simulink model "templatePQVFreplay"  (R2019b)
settings: Solver=ode23t  StartTime=0  StopTime=dataSim(l).Time(end)  FixedStep=Ts
model workspace (MAT data in the model file):
  AC8B_test_sdosession : sldodialogs.data.SessionData (value not decoded)
  tp34291882_bceb_4da8_b486_81ba615ab517 = [0 0.0333333 0.0666667 0.1 0.1333334 0.1666667 0.2 0.2333333 0.2666666 0.2999999 0.3333332 0.3666665 ... (13500 elements, 2700x5)]
  tp5fd81924_c6b2_4820_a4c1_c746ac51258e : object (value not decoded)
  tp61e2f470_2812_498a_af75_e87b8b944307 = [0 0.0333333 0.0666667 0.1 0.1333334 0.1666667 0.2 0.2333333 0.2666666 0.2999999 0.3333332 0.3666665 ... (13500 elements, 2700x5)]
  tpfa3056f0_c430_45b3_969f_b76cef1498ad : object (value not decoded)
undefined symbols (not defined in the file): dataSim, Fnom, l, MBase, Psnubber, Rsnubber, sys, Vnom
libraries: modelLibrary x8, powerlib x4, powerlib_meascontrol x1, GenLib x1, ideal_source x1
(part 2 of 2)

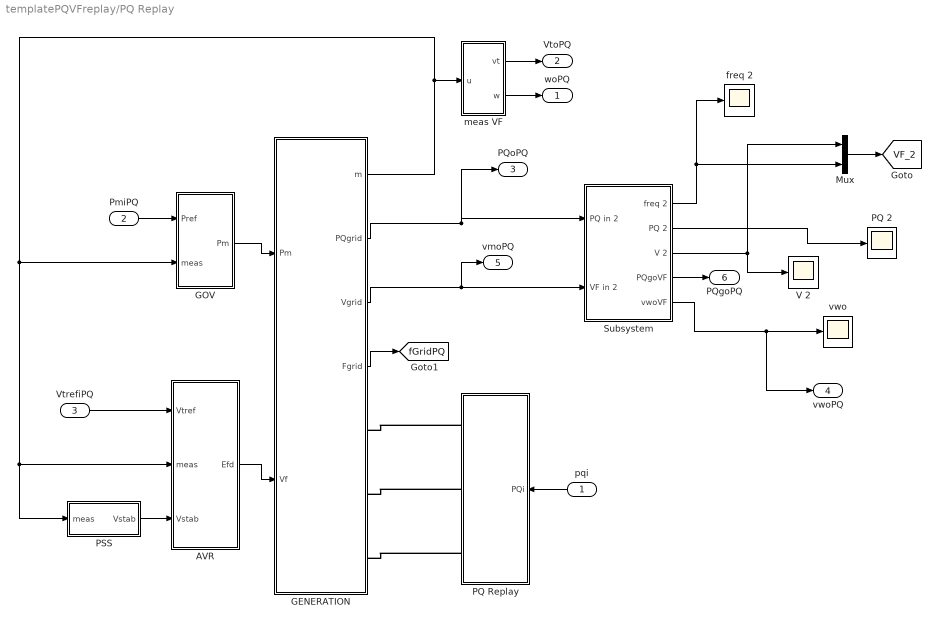
== system templatePQVFreplay/PQ Replay ==
  pqi : Inport  PortDimensions=2
  PmiPQ : Inport  Port=2
  VtrefiPQ : Inport  Port=3
  AVR : Subsystem  BlockChoice=ST4B
      link override ST4B: p=dyn.exst4b_31923_COLUSGT1
      settings: AttributesFormatString=%<BlockChoice>  TemplateBlock=modelLibrary/AVR  MemberBlocks=REXS,ST1A,ST4B
  GENERATION : Subsystem  BlockChoice=GENTPJ_TERMINAL
      link override GENROU_TERMINAL: g=sys.GENERATOR(1)  p=dyn.genrou_31923_COLUSGT1
      link override GENTPJ_TERMINAL: g=sys.GENERATOR(1)  p=dyn.genrou_31923_COLUSGT1
      settings: AttributesFormatString=%<BlockChoice>  TemplateBlock=modelLibrary/GENERATION  MemberBlocks=GENROU_TERMINAL,GENROU_TRANSFORMER,GENSAL_TRANSFORMER,GENTPJ_TERMINAL,GENTPJ_TRANSFORMER
  GOV : Subsystem  BlockChoice=GGOV1
      link override GGOV1: p=dyn.ggov1_31923_COLUSGT1  g=sys.GENERATOR(2)
      settings: AttributesFormatString=%<BlockChoice>  TemplateBlock=modelLibrary/GOV  MemberBlocks=GGOV1,IEEEG3
  Mux : Mux  Inputs=2
  PQ 2 : Scope
  PQ Replay : Subsystem  mask{Vrms=dataSim.Vact(1)*1e3, FreqHz=dataSim.Fact(1)}
      mask prompts: Vrms "Nominal LL Voltage (RMS)"; FreqHz "Frequency (Hz)"
  PSS : Subsystem  BlockChoice=PSS2B
      link override PSS2B: p=dyn.pss2b_31923_COLUSGT1
      link override PSS2B/Bus Selector3: OutputSignals="Mechanical.Rotor speed deviation  dw (pu),Mechanical.Electrical power  Pe (pu)"
      settings: AttributesFormatString=%<BlockChoice>  TemplateBlock=modelLibrary/PSS  MemberBlocks=PSS1A,PSS2A,PSS2B
  Subsystem : Subsystem
  V 2 : Scope
  freq 2 : Scope
  meas VF : Subsystem
  vwo : Scope
  woPQ : Outport
  VtoPQ : Outport  Port=2
  PQoPQ : Outport  Port=3  SampleTime=1/30
  vwoPQ : Outport  Port=4
  vmoPQ : Outport  Port=5
  PQgoPQ : Outport  Port=6  SampleTime=1/30
  tag scope: VF_2=global, fGridPQ=global
  wires:
  GENERATION/3(Vgrid) -> vmoPQ/1, Subsystem/2(VF in 2)
  GENERATION/1(m) -> GOV/2(meas), PSS/1(meas), AVR/2(meas), meas VF/1(u)
  GENERATION/2(PQgrid) -> PQoPQ/1, Subsystem/1(PQ in 2)
  meas VF/1(vt) -> VtoPQ/1
  meas VF/2(w) -> woPQ/1
  Subsystem/1(freq 2) -> Mux/2, freq 2/1
  Subsystem/2(PQ 2) -> PQ 2/1
  Subsystem/4(PQgoVF) -> PQgoPQ/1
  Subsystem/3(V 2) -> V 2/1, Mux/1
  Subsystem/5(vwoVF) -> vwoPQ/1, vwo/1
  PmiPQ/1 -> GOV/1(Pref)
  GOV/1(Pm) -> GENERATION/1(Pm)
  AVR/1(Efd) -> GENERATION/2(Vf)
  VtrefiPQ/1 -> AVR/1(Vtref)
  pqi/1 -> PQ Replay/1(PQi)
  PSS/1(Vstab) -> AVR/3(Vstab)
  Mux/1 -> [VF_2]
  GENERATION/4(Fgrid) -> [fGridPQ]
  connections:
  PQ Replay/RConn1 -- GENERATION/RConn1
  PQ Replay/RConn2 -- GENERATION/RConn2
  PQ Replay/RConn3 -- GENERATION/RConn3

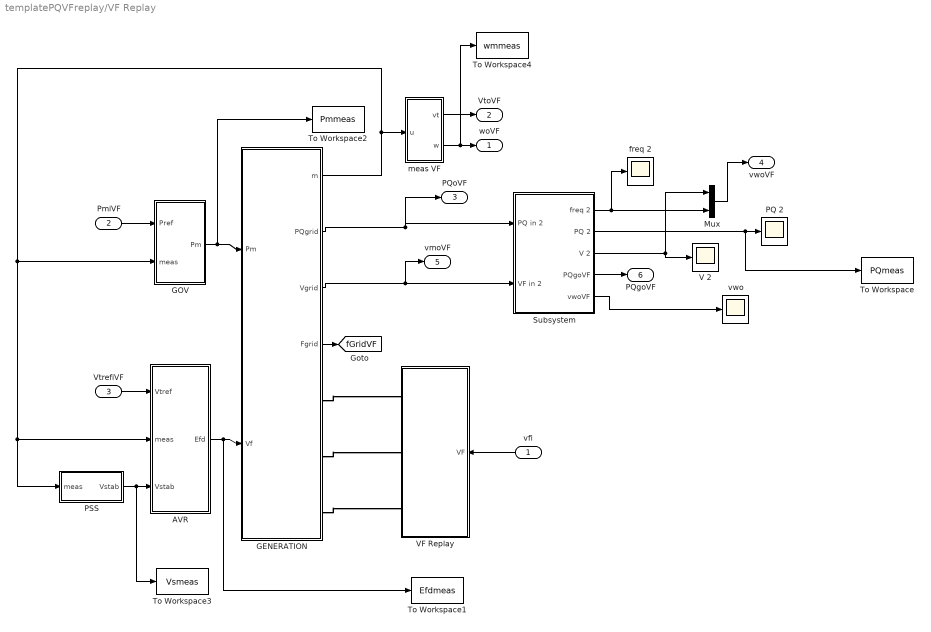
== system templatePQVFreplay/VF Replay ==
  vfi : Inport  PortDimensions=2
  PmiVF : Inport  Port=2
  VtrefiVF : Inport  Port=3
  AVR : Subsystem  BlockChoice=ST4B
      link override ST4B: p=dyn.exst4b_31923_COLUSGT1
      settings: AttributesFormatString=%<BlockChoice>  TemplateBlock=modelLibrary/AVR  MemberBlocks=REXS,ST1A,ST4B
  GENERATION : Subsystem  BlockChoice=GENTPJ_TERMINAL
      link override GENROU_TERMINAL: g=sys.GENERATOR(1)  p=dyn.genrou_31923_COLUSGT1
      link override GENTPJ_TERMINAL: g=sys.GENERATOR(1)  p=dyn.genrou_31923_COLUSGT1
      settings: AttributesFormatString=%<BlockChoice>  TemplateBlock=modelLibrary/GENERATION  MemberBlocks=GENROU_TERMINAL,GENROU_TRANSFORMER,GENSAL_TRANSFORMER,GENTPJ_TERMINAL,GENTPJ_TRANSFORMER
  GOV : Subsystem  BlockChoice=GGOV1
      link override GGOV1: p=dyn.ggov1_31923_COLUSGT1  g=sys.GENERATOR(2)
      settings: AttributesFormatString=%<BlockChoice>  TemplateBlock=modelLibrary/GOV  MemberBlocks=GGOV1,IEEEG3
  Mux : Mux  Inputs=2
  PQ 2 : Scope
  PSS : Subsystem  BlockChoice=PSS2B
      link override PSS2B: p=dyn.pss2b_31923_COLUSGT1
      link override PSS2B/Bus Selector3: OutputSignals="Mechanical.Rotor speed deviation  dw (pu),Mechanical.Electrical power  Pe (pu)"
      settings: AttributesFormatString=%<BlockChoice>  TemplateBlock=modelLibrary/PSS  MemberBlocks=PSS1A,PSS2A,PSS2B
  Subsystem : Subsystem
  To Workspace : ToWorkspace  VariableName=PQmeas  SampleTime=1/60
  To Workspace1 : ToWorkspace  VariableName=Efdmeas  SampleTime=1/60
  To Workspace2 : ToWorkspace  VariableName=Pmmeas  SampleTime=1/60
  To Workspace3 : ToWorkspace  VariableName=Vsmeas  SampleTime=1/60
  To Workspace4 : ToWorkspace  VariableName=wmmeas  SampleTime=1/60
  V 2 : Scope
  VF Replay : Subsystem
  freq 2 : Scope
  meas VF : Subsystem
  vwo : Scope
  woVF : Outport
  VtoVF : Outport  Port=2
  PQoVF : Outport  Port=3  SampleTime=1/30
  vwoVF : Outport  Port=4
  vmoVF : Outport  Port=5
  PQgoVF : Outport  Port=6  SampleTime=1/30
  tag scope: fGridVF=global
  wires:
  GENERATION/3(Vgrid) -> vmoVF/1, Subsystem/2(VF in 2)
  GENERATION/2(PQgrid) -> PQoVF/1, Subsystem/1(PQ in 2)
  meas VF/1(vt) -> VtoVF/1
  Subsystem/1(freq 2) -> freq 2/1, Mux/2
  Subsystem/2(PQ 2) -> To Workspace/1, PQ 2/1
  Subsystem/4(PQgoVF) -> PQgoVF/1
  Subsystem/3(V 2) -> V 2/1, Mux/1
  Subsystem/5(vwoVF) -> vwo/1
  Mux/1 -> vwoVF/1
  PmiVF/1 -> GOV/1(Pref)
  GOV/1(Pm) -> To Workspace2/1, GENERATION/1(Pm)
  PSS/1(Vstab) -> To Workspace3/1, AVR/3(Vstab)
  AVR/1(Efd) -> To Workspace1/1, GENERATION/2(Vf)
  VtrefiVF/1 -> AVR/1(Vtref)
  vfi/1 -> VF Replay/1(VF)
  GENERATION/1(m) -> GOV/2(meas), PSS/1(meas), AVR/2(meas), meas VF/1(u)
  meas VF/2(w) -> To Workspace4/1, woVF/1
  GENERATION/4(Fgrid) -> [fGridVF]
  connections:
  GENERATION/RConn1 -- VF Replay/RConn1
  GENERATION/RConn2 -- VF Replay/RConn2
  GENERATION/RConn3 -- VF Replay/RConn3

== system templatePQVFreplay/view ==
  Gain : Gain  Gain=1/MBase
  Selector2 : Selector  InputPortWidth=4  IndexOptions=Index vector (dialog)  Indices=[2 4]  OutputSizes=1
  Selector3 : Selector  InputPortWidth=4  IndexOptions=Index vector (dialog)  Indices=[1 3]  OutputSizes=1
  P : Outport
  Q : Outport  Port=2
  wires:
  [PQ_2] -> Gain/1
  Gain/1 -> Selector2/1, Selector3/1
  Selector2/1 -> Q/1
  Selector3/1 -> P/1

== system templatePQVFreplay/view1 ==
  Gain : Gain
  Selector2 : Selector  InputPortWidth=4  IndexOptions=Index vector (dialog)  Indices=[3 4]  OutputSizes=1
  Selector3 : Selector  InputPortWidth=4  IndexOptions=Index vector (dialog)  Indices=[1 2]  OutputSizes=1
  V : Outport
  F : Outport  Port=2
  wires:
  [VF_2] -> Gain/1
  Gain/1 -> Selector2/1, Selector3/1
  Selector2/1 -> F/1
  Selector3/1 -> V/1

== system templatePQVFreplay/PQ Replay/AVR ==
  Vtref : Inport
  meas : Inport  Port=2
  Vstab : Inport  Port=3
  ST4B : modelLibrary/ST4B  p=dyn.exst4b_31923_COLUSGT1
  Efd : Outport
  wires:
  Vtref/1 -> ST4B/1
  meas/1 -> ST4B/2
  Vstab/1 -> ST4B/3
  ST4B/1 -> Efd/1

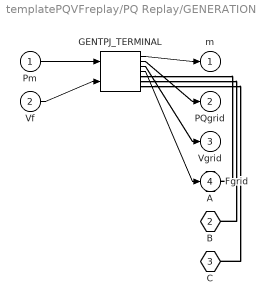
== system templatePQVFreplay/PQ Replay/GENERATION ==
  Pm : Inport
  Vf : Inport  Port=2
  GENTPJ_TERMINAL : modelLibrary/GENTPJ_TERMINAL  g=sys.GENERATOR(1)  p=dyn.genrou_31923_COLUSGT1
  A : PMIOPort  Side=Right
  B : PMIOPort  Port=2  Side=Right
  C : PMIOPort  Port=3  Side=Right
  m : Outport
  PQgrid : Outport  Port=2
  Vgrid : Outport  Port=3
  Fgrid : Outport  Port=4
  wires:
  Pm/1 -> GENTPJ_TERMINAL/1
  Vf/1 -> GENTPJ_TERMINAL/2
  GENTPJ_TERMINAL/1 -> m/1
  GENTPJ_TERMINAL/2 -> PQgrid/1
  GENTPJ_TERMINAL/3 -> Vgrid/1
  GENTPJ_TERMINAL/4 -> Fgrid/1
  connections:
  GENTPJ_TERMINAL/RConn1 -- A/RConn1
  GENTPJ_TERMINAL/RConn2 -- B/RConn1
  GENTPJ_TERMINAL/RConn3 -- C/RConn1

== system templatePQVFreplay/PQ Replay/GOV ==
  Pref : Inport
  meas : Inport  Port=2
  GGOV1 : modelLibrary/GGOV1  p=dyn.ggov1_31923_COLUSGT1  g=sys.GENERATOR(2)
  Pm : Outport
  wires:
  Pref/1 -> GGOV1/1
  meas/1 -> GGOV1/2
  GGOV1/1 -> Pm/1

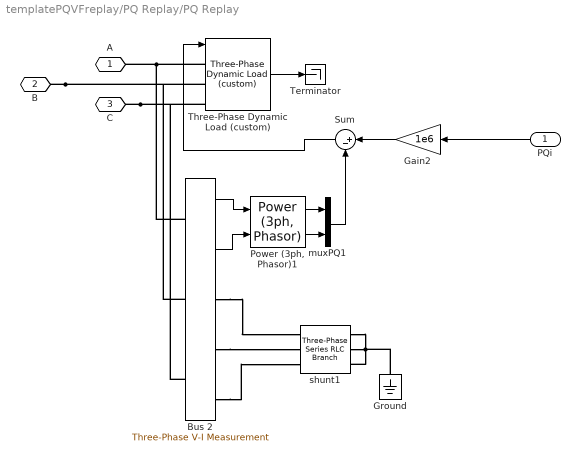
== system templatePQVFreplay/PQ Replay/PQ Replay ==
  PQi : Inport
  Bus 2 : powerlib/Measurements/Three-Phase V-I Measurement  VoltageMeasurement=phase-to-ground  SetLabelV=off  LabelV=Vabc  Vpu=off  VpuLL=off  CurrentMeasurement=yes  SetLabelI=off  LabelI=Iabc  Ipu=off  Pbase=100e6  Vbase=500e3  OutputType=Complex  PhasorSimulation=on  PSBequivalent=0
      settings: SourceProductName=Simscape Electrical
  Gain2 : Gain  Gain=1e6
  Ground : powerlib/Elements/Ground  LConnTagsString=a
      settings: SourceProductName=Simscape Electrical
  "Power (3ph, Phasor)1" : powerlib_meascontrol/Measurements/Power (3ph, Phasor)
      settings: SourceProductName=Simscape Electrical  SourceProductBaseCode=PS
  Sum : Sum  Inputs=|+-
  Terminator : Terminator
  Three-Phase Dynamic Load (custom) : GenLib/Three-Phase Dynamic Load (custom)  NominalVoltage=[ Vrms FreqHz ]  ActiveReactivePowers="[-dataSim.Pact(1)-Psnubber/1e6  -dataSim.Qact(1)]*1e6"  PositiveSequence=[1 0]  ExternalControl=on  NpNq=[1.3 2]  TimeConstants="[0  0  0  0]"  MinimumVoltage=0.7  LoadFlowParameters=[4,0,0,0,0]
  muxPQ1 : Mux  Inputs=2
  shunt1 : powerlib/Elements/Three-Phase Series RLC Branch  LConnTagsString=A|B|C  RConnTagsString=A|B|C  BranchType=R  Resistance=Rsnubber  Inductance=1e-3  Capacitance=1e-6  Measurements=None
      settings: SourceProductName=Simscape Electrical
  A : PMIOPort  Side=Right
  B : PMIOPort  Port=2  Side=Right
  C : PMIOPort  Port=3  Side=Right
  wires:
  Three-Phase Dynamic Load (custom)/1 -> Terminator/1
  Bus 2/2 -> "Power (3ph, Phasor)1"/2
  Bus 2/1 -> "Power (3ph, Phasor)1"/1
  Sum/1 -> Three-Phase Dynamic Load (custom)/1
  "Power (3ph, Phasor)1"/2 -> muxPQ1/2
  Gain2/1 -> Sum/1
  "Power (3ph, Phasor)1"/1 -> muxPQ1/1
  PQi/1 -> Gain2/1
  muxPQ1/1 -> Sum/2
  connections:
  B/RConn1 -- Three-Phase Dynamic Load (custom)/LConn2 -- Bus 2/LConn2
  Bus 2/LConn1 -- Three-Phase Dynamic Load (custom)/LConn1 -- A/RConn1
  C/RConn1 -- Three-Phase Dynamic Load (custom)/LConn3 -- Bus 2/LConn3
  Bus 2/RConn1 -- shunt1/LConn1
  Bus 2/RConn2 -- shunt1/LConn2
  Bus 2/RConn3 -- shunt1/LConn3
  shunt1/RConn1 -- shunt1/RConn2 -- Ground/LConn1 -- shunt1/RConn3

== system templatePQVFreplay/PQ Replay/PSS ==
  meas : Inport
  PSS2B : modelLibrary/PSS2B  p=dyn.pss2b_31923_COLUSGT1
  Vstab : Outport
  wires:
  meas/1 -> PSS2B/1
  PSS2B/1 -> Vstab/1

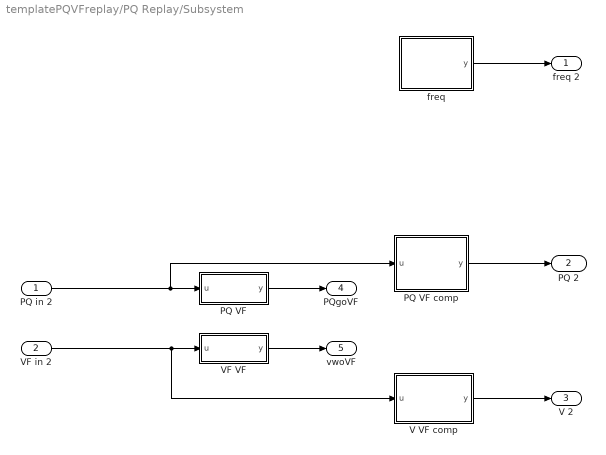
== system templatePQVFreplay/PQ Replay/Subsystem ==
  PQ in 2 : Inport
  VF in 2 : Inport  Port=2
  PQ VF : Subsystem
  PQ VF comp : Subsystem
  V VF comp : Subsystem
  VF VF : Subsystem
  freq : Subsystem
  freq 2 : Outport
  PQ 2 : Outport  Port=2
  V 2 : Outport  Port=3
  PQgoVF : Outport  Port=4
  vwoVF : Outport  Port=5
  wires:
  V VF comp/1(y) -> V 2/1
  VF in 2/1 -> V VF comp/1(u), VF VF/1(u)
  PQ VF comp/1("y ") -> PQ 2/1
  freq/1(y) -> freq 2/1
  PQ VF/1(y) -> PQgoVF/1
  VF VF/1(y) -> vwoVF/1
  PQ in 2/1 -> PQ VF/1(u), PQ VF comp/1(u)

== system templatePQVFreplay/PQ Replay/meas VF ==
  u : Inport
  Bus Selector6 : BusSelector  OutputSignals="dq0 components.Stator voltage  vd (pu),dq0 components.Stator voltage  vq (pu),Mechanical.Rotor speed  wm  (pu)"
  Euclidian Norm5 : Subsystem
  wo PQ : Subsystem
  vt : Outport
  w : Outport  Port=2
  wires:
  u/1 -> Bus Selector6/1
  Bus Selector6/2 -> Euclidian Norm5/2(u2)  "<Stator voltage  vq (pu)>"
  Bus Selector6/1 -> Euclidian Norm5/1(u1)  "<Stator voltage  vd (pu)>"
  Euclidian Norm5/1(y) -> vt/1  "vt"
  Bus Selector6/3 -> wo PQ/1(u)  "<Rotor speed  wm  (pu)>"
  wo PQ/1(y) -> w/1

== system templatePQVFreplay/VF Replay/AVR ==
  Vtref : Inport
  meas : Inport  Port=2
  Vstab : Inport  Port=3
  ST4B : modelLibrary/ST4B  p=dyn.exst4b_31923_COLUSGT1
  Efd : Outport
  wires:
  Vtref/1 -> ST4B/1
  meas/1 -> ST4B/2
  Vstab/1 -> ST4B/3
  ST4B/1 -> Efd/1

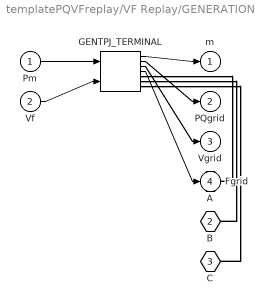
== system templatePQVFreplay/VF Replay/GENERATION ==
  Pm : Inport
  Vf : Inport  Port=2
  GENTPJ_TERMINAL : modelLibrary/GENTPJ_TERMINAL  g=sys.GENERATOR(1)  p=dyn.genrou_31923_COLUSGT1
  A : PMIOPort  Side=Right
  B : PMIOPort  Port=2  Side=Right
  C : PMIOPort  Port=3  Side=Right
  m : Outport
  PQgrid : Outport  Port=2
  Vgrid : Outport  Port=3
  Fgrid : Outport  Port=4
  wires:
  Pm/1 -> GENTPJ_TERMINAL/1
  Vf/1 -> GENTPJ_TERMINAL/2
  GENTPJ_TERMINAL/1 -> m/1
  GENTPJ_TERMINAL/2 -> PQgrid/1
  GENTPJ_TERMINAL/3 -> Vgrid/1
  GENTPJ_TERMINAL/4 -> Fgrid/1
  connections:
  GENTPJ_TERMINAL/RConn1 -- A/RConn1
  GENTPJ_TERMINAL/RConn2 -- B/RConn1
  GENTPJ_TERMINAL/RConn3 -- C/RConn1

== system templatePQVFreplay/VF Replay/GOV ==
  Pref : Inport
  meas : Inport  Port=2
  GGOV1 : modelLibrary/GGOV1  p=dyn.ggov1_31923_COLUSGT1  g=sys.GENERATOR(2)
  Pm : Outport
  wires:
  Pref/1 -> GGOV1/1
  meas/1 -> GGOV1/2
  GGOV1/1 -> Pm/1

== system templatePQVFreplay/VF Replay/PSS ==
  meas : Inport
  PSS2B : modelLibrary/PSS2B  p=dyn.pss2b_31923_COLUSGT1
  Vstab : Outport
  wires:
  meas/1 -> PSS2B/1
  PSS2B/1 -> Vstab/1

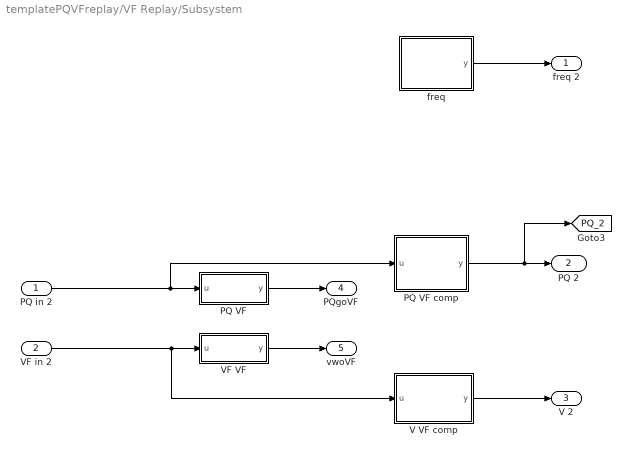
== system templatePQVFreplay/VF Replay/Subsystem ==
  PQ in 2 : Inport
  VF in 2 : Inport  Port=2
  PQ VF : Subsystem
  PQ VF comp : Subsystem
  V VF comp : Subsystem
  VF VF : Subsystem
  freq : Subsystem
  freq 2 : Outport
  PQ 2 : Outport  Port=2
  V 2 : Outport  Port=3
  PQgoVF : Outport  Port=4
  vwoVF : Outport  Port=5
  tag scope: PQ_2=global
  wires:
  V VF comp/1(y) -> V 2/1
  VF in 2/1 -> V VF comp/1(u), VF VF/1(u)
  PQ VF comp/1("y ") -> [PQ_2], PQ 2/1
  freq/1(y) -> freq 2/1
  PQ VF/1(y) -> PQgoVF/1
  VF VF/1(y) -> vwoVF/1
  PQ in 2/1 -> PQ VF/1(u), PQ VF comp/1(u)

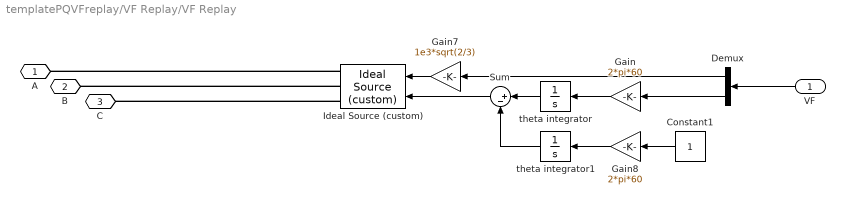
== system templatePQVFreplay/VF Replay/VF Replay ==
  VF : Inport
  Constant1 : Constant
  Demux : Demux  Outputs=2
  Gain : Gain  Gain=2*pi*60
  Gain7 : Gain  Gain=1e3*sqrt(2/3)
  Gain8 : Gain  Gain=2*pi*60
  Ideal Source (custom) : ideal_source/Ideal Source (custom)  InternalConnection=Yg  VoltagePhases=off  Voltage=sys.BUS(1).VBUS*1e3  PhaseAngle=0  Voltage_phases=[25e3 25e3 25e3]/sqrt(3)  PhaseAngles_phases=[0 -120 +120]  Frequency=60  NonIdealSource=on  SpecifyImpedance=off  Resistance=1e-5  Inductance=1e-5  ShortCircuitLevel=100e6  BaseVoltage=sys.BUS(1).VBUS*1e3  XRratio=7  BusType=swing  Pref=10e3  Qref=0  Prefabc=[10e3, 10e3, 10e3]  Qrefabc=[0, 0, 0]  Qmin=-inf  Qmax=inf
  Sum : Sum  Inputs=|+-
  theta integrator : Integrator  InitialCondition=2*pi*60
  theta integrator1 : Integrator  InitialCondition=2*pi*60
  A : PMIOPort  Side=Right
  B : PMIOPort  Port=2  Side=Right
  C : PMIOPort  Port=3  Side=Right
  wires:
  theta integrator/1 -> Sum/1
  Constant1/1 -> Gain8/1
  Gain7/1 -> Ideal Source (custom)/2
  VF/1 -> Demux/1
  Demux/2 -> Gain/1
  Gain/1 -> theta integrator/1
  Sum/1 -> Ideal Source (custom)/1
  Demux/1 -> Gain7/1
  theta integrator1/1 -> Sum/2
  Gain8/1 -> theta integrator1/1
  connections:
  Ideal Source (custom)/RConn2 -- B/RConn1
  Ideal Source (custom)/RConn1 -- C/RConn1
  Ideal Source (custom)/RConn3 -- A/RConn1

== system templatePQVFreplay/VF Replay/meas VF ==
  u : Inport
  Bus Selector6 : BusSelector  OutputSignals="dq0 components.Stator voltage  vd (pu),dq0 components.Stator voltage  vq (pu),Mechanical.Rotor speed  wm  (pu)"
  Euclidian Norm5 : Subsystem
  wo VF : Subsystem
  vt : Outport
  w : Outport  Port=2
  wires:
  u/1 -> Bus Selector6/1
  Bus Selector6/2 -> Euclidian Norm5/2(u2)  "<Stator voltage  vq (pu)>"
  Bus Selector6/1 -> Euclidian Norm5/1(u1)  "<Stator voltage  vd (pu)>"
  Euclidian Norm5/1(y) -> vt/1  "vt"
  Bus Selector6/3 -> wo VF/1(u)  "<Rotor speed  wm  (pu)>"
  wo VF/1(y) -> w/1

== system templatePQVFreplay/PQ Replay/Subsystem/PQ VF ==
  u : Inport
  Constant1 : Constant  Value=[dataSim(l).Pact(1) dataSim(l).Qact(1)]
  GainPQgo : Gain  Gain=[1/dataSim(l).maxP 1/dataSim(l).maxQ]
  Sum1 : Sum  Inputs=|+-
  y : Outport  SampleTime=1/30
  wires:
  u/1 -> Sum1/1
  GainPQgo/1 -> y/1
  Sum1/1 -> GainPQgo/1
  Constant1/1 -> Sum1/2

== system templatePQVFreplay/PQ Replay/Subsystem/PQ VF comp ==
  u : Inport
  From Workspace3 : FromWorkspace  VariableName=[dataSim(l).Time dataSim(l).Pact dataSim(l).Qact]  SampleTime=0
  Mux2 : Mux  Inputs=2
  "y " : Outport
  wires:
  u/1 -> Mux2/2
  Mux2/1 -> "y "/1
  From Workspace3/1 -> Mux2/1

== system templatePQVFreplay/PQ Replay/Subsystem/V VF comp ==
  u : Inport
  From Workspace5 : FromWorkspace  VariableName=[dataSim(l).Time dataSim(l).Vact]  SampleTime=0
  Mux6 : Mux  Inputs=2
  To File5 : ToFile  Filename=vsVF.mat  MatrixName=vVF  SaveFormat=Timeseries
  y : Outport
  wires:
  u/1 -> Mux6/2
  From Workspace5/1 -> Mux6/1
  Mux6/1 -> y/1, To File5/1

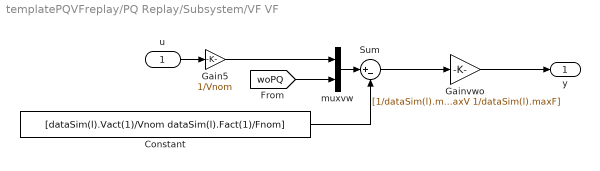
== system templatePQVFreplay/PQ Replay/Subsystem/VF VF ==
  u : Inport
  Constant : Constant  Value=[dataSim(l).Vact(1)/Vnom dataSim(l).Fact(1)/Fnom]
  Gain5 : Gain  Gain=1/Vnom
  Gainvwo : Gain  Gain=[1/dataSim(l).maxV 1/dataSim(l).maxF]
  Sum : Sum  Inputs=|+-
  muxvw : Mux  Inputs=2
  y : Outport
  wires:
  u/1 -> Gain5/1
  Gainvwo/1 -> y/1
  Gain5/1 -> muxvw/1
  muxvw/1 -> Sum/1
  Constant/1 -> Sum/2
  Sum/1 -> Gainvwo/1
  [woPQ] -> muxvw/2

== system templatePQVFreplay/PQ Replay/Subsystem/freq ==
  From Workspace4 : FromWorkspace  VariableName=[dataSim(l).Time dataSim(l).Fact/Fnom]  SampleTime=0
  Mux5 : Mux  Inputs=2
  y : Outport
  wires:
  Mux5/1 -> y/1
  From Workspace4/1 -> Mux5/1
  [fGridPQ] -> Mux5/2

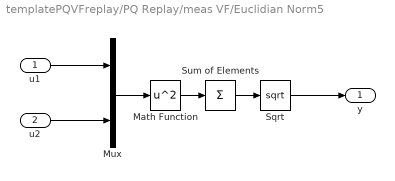
== system templatePQVFreplay/PQ Replay/meas VF/Euclidian Norm5 ==
  u1 : Inport
  u2 : Inport  Port=2
  Math Function : Math  Operator=square  SaturateOnIntegerOverflow=on
  Mux : Mux  Inputs=2
  Sqrt : Sqrt  SaturateOnIntegerOverflow=on
  Sum of Elements : Sum  Inputs=+
  y : Outport
  wires:
  Sqrt/1 -> y/1
  Mux/1 -> Math Function/1
  u2/1 -> Mux/2
  u1/1 -> Mux/1
  Math Function/1 -> Sum of Elements/1
  Sum of Elements/1 -> Sqrt/1

== system templatePQVFreplay/PQ Replay/meas VF/wo PQ ==
  u : Inport
  Gainwo : Gain
  y : Outport
  tag scope: woPQ=global
  wires:
  u/1 -> Gainwo/1
  Gainwo/1 -> [woPQ], y/1

== system templatePQVFreplay/VF Replay/Subsystem/PQ VF ==
  u : Inport
  Constant1 : Constant  Value=[dataSim(l).Pact(1) dataSim(l).Qact(1)]
  GainPQgo : Gain  Gain=[1/dataSim(l).maxP 1/dataSim(l).maxQ]
  Sum1 : Sum  Inputs=|+-
  y : Outport  SampleTime=1/30
  tag scope: PQgoVF=global
  wires:
  u/1 -> Sum1/1
  GainPQgo/1 -> [PQgoVF], y/1
  Sum1/1 -> GainPQgo/1
  Constant1/1 -> Sum1/2

== system templatePQVFreplay/VF Replay/Subsystem/PQ VF comp ==
  u : Inport
  From Workspace3 : FromWorkspace  VariableName=[dataSim(l).Time dataSim(l).Pact dataSim(l).Qact]  SampleTime=0
  Mux2 : Mux  Inputs=2
  To File4 : ToFile  Filename=PQsVF.mat  MatrixName=PQVF  SaveFormat=Timeseries  SampleTime=1/30
  "y " : Outport
  wires:
  u/1 -> Mux2/2
  Mux2/1 -> "y "/1, To File4/1
  From Workspace3/1 -> Mux2/1

== system templatePQVFreplay/VF Replay/Subsystem/V VF comp ==
  u : Inport
  From Workspace5 : FromWorkspace  VariableName=[dataSim(l).Time dataSim(l).Vact]  SampleTime=0
  Mux6 : Mux  Inputs=2
  y : Outport
  wires:
  u/1 -> Mux6/2
  From Workspace5/1 -> Mux6/1
  Mux6/1 -> y/1

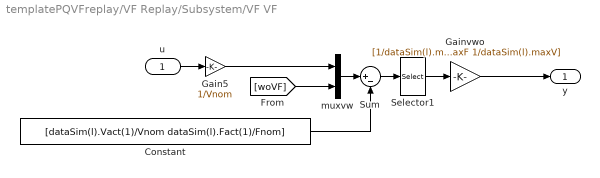
== system templatePQVFreplay/VF Replay/Subsystem/VF VF ==
  u : Inport
  Constant : Constant  Value=[dataSim(l).Vact(1)/Vnom dataSim(l).Fact(1)/Fnom]
  Gain5 : Gain  Gain=1/Vnom
  Gainvwo : Gain  Gain=[1/dataSim(l).maxF 1/dataSim(l).maxV]
  Selector1 : Selector  InputPortWidth=2  IndexOptions=Index vector (dialog)  Indices=[2 1]  OutputSizes=1
  Sum : Sum  Inputs=|+-
  muxvw : Mux  Inputs=2
  y : Outport
  wires:
  u/1 -> Gain5/1
  Gainvwo/1 -> y/1
  Gain5/1 -> muxvw/1
  Sum/1 -> Selector1/1
  muxvw/1 -> Sum/1
  Constant/1 -> Sum/2
  Selector1/1 -> Gainvwo/1
  [woVF] -> muxvw/2

== system templatePQVFreplay/VF Replay/Subsystem/freq ==
  From Workspace4 : FromWorkspace  VariableName=[dataSim(l).Time dataSim(l).Fact/Fnom]  SampleTime=0
  Mux5 : Mux  Inputs=2
  To File3 : ToFile  Filename=wsVF.mat  MatrixName=wVF  SaveFormat=Timeseries
  y : Outport
  wires:
  Mux5/1 -> y/1, To File3/1
  From Workspace4/1 -> Mux5/1
  [fGridVF] -> Mux5/2

== system templatePQVFreplay/VF Replay/meas VF/Euclidian Norm5 ==
  u1 : Inport
  u2 : Inport  Port=2
  Math Function : Math  Operator=square  SaturateOnIntegerOverflow=on
  Mux : Mux  Inputs=2
  Sqrt : Sqrt  SaturateOnIntegerOverflow=on
  Sum of Elements : Sum  Inputs=+
  y : Outport
  wires:
  Sqrt/1 -> y/1
  Mux/1 -> Math Function/1
  u2/1 -> Mux/2
  u1/1 -> Mux/1
  Math Function/1 -> Sum of Elements/1
  Sum of Elements/1 -> Sqrt/1

== system templatePQVFreplay/VF Replay/meas VF/wo VF ==
  u : Inport
  Gainwo : Gain
  y : Outport
  wires:
  u/1 -> Gainwo/1
  Gainwo/1 -> y/1
